simulink model "Guardian_Battery"  (R2025b)
settings: Solver=FixedStepDiscrete  StartTime=0.0  StopTime=T_end_s  FixedStep=Ts  RelTol=1e-3
model workspace (MAT data in the model file):
  TLS_impl_select = 2
values from neighbouring files (symbols this model uses):
  a1_coef = exp(-Ts/(tau1_s))    [Guardian_Battery_script.m]
  a2_coef = exp(-Ts/(tau2_s))    [Guardian_Battery_script.m]
  hyst_filt_den = [1, -a_hyst_coef]    [Guardian_Battery_script.m]
  hyst_filt_num = 1 - a_hyst_coef    (= 0.00201823135843)    [Guardian_Battery_script.m]
  OCV_data = ocvLookupTbl.OCV_V    [Guardian_Battery_script.m]
  Q_nominal = 50    [Guardian_Battery_script.m]
  R0_ref = 0.0007    [Guardian_Battery_script.m]
  R1_ref = 0.0016    [Guardian_Battery_script.m]
  R2_ref = 0.00035    [Guardian_Battery_script.m]
  SOC_breakpoints = ocvLookupTbl.SOC_pct    [Guardian_Battery_script.m]
  SOC_init_pct = 80    [Guardian_Battery_script.m]
  Ts = 0.1    [Guardian_Battery_script.m]
undefined symbols (not defined in the file or in its folder): DiscIntNeverNeededParam, dspblkCoreblockFVToolHelper, gcbh
libraries: simulink x2
settings Model: Creator=LENOVO  LastModifiedBy=Ahmed

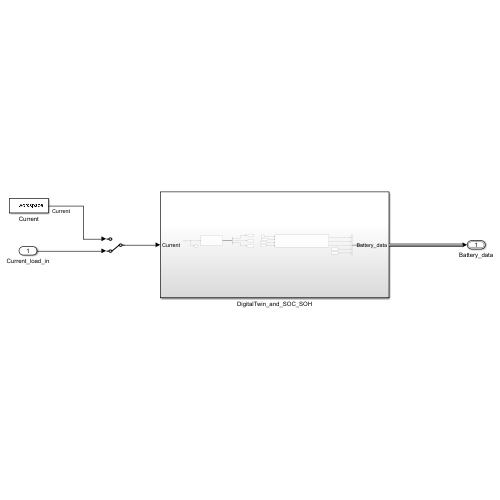
[thumbnail: Simulink's stored preview of the top-level diagram]
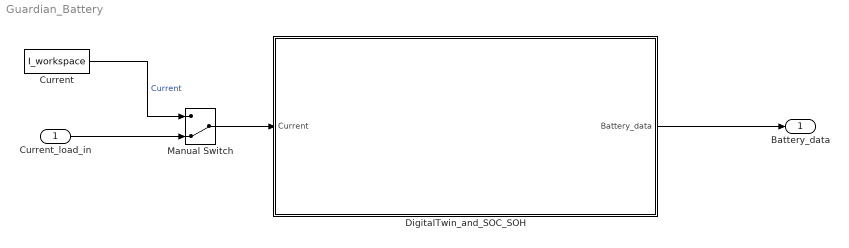
== system Guardian_Battery ==
  Current_load_in : Inport
  Current : FromWorkspace  VariableName=I_workspace
  DigitalTwin_and_SOC_SOH : Subsystem
  Manual Switch : ManualSwitch  CurrentSetting=0
  Battery_data : Outport  OutDataTypeStr=Bus: BatteryDataBus
  wires:
  DigitalTwin_and_SOC_SOH/1(Battery_data) -> Battery_data/1
  Current/1 -> Manual Switch/1  "Current"
  Manual Switch/1 -> DigitalTwin_and_SOC_SOH/1(Current)
  Current_load_in/1 -> Manual Switch/2

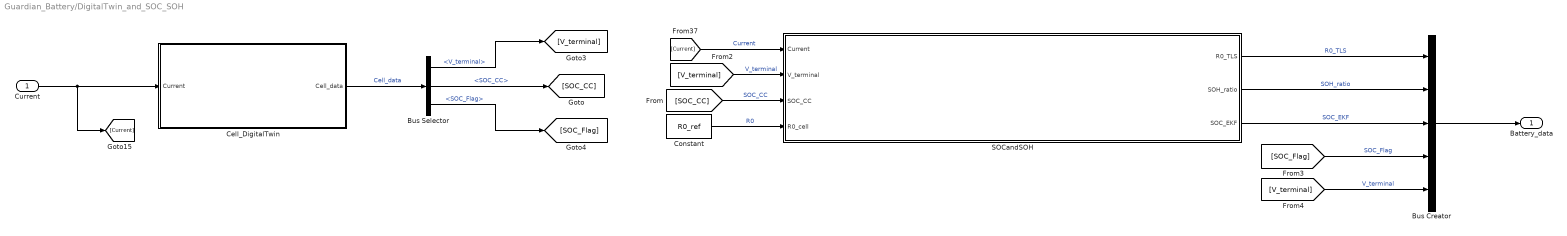
== system Guardian_Battery/DigitalTwin_and_SOC_SOH ==
  Current : Inport
  Bus Creator : BusCreator  Inputs=5  OutDataTypeStr=Bus: BatteryDataBus
  Bus Selector : BusSelector  OutputSignals=V_terminal,SOC_CC,SOC_Flag
  Cell_DigitalTwin : Subsystem
  Constant : Constant  Value=R0_ref
  SOCandSOH : Subsystem
  Battery_data : Outport  OutDataTypeStr=Bus: BatteryDataBus
  wires:
  Bus Selector/1 -> [V_terminal]  "<V_terminal>"
  Bus Selector/2 -> [SOC_CC]  "<SOC_CC>"
  Bus Selector/3 -> [SOC_Flag]  "<SOC_Flag>"
  Cell_DigitalTwin/1(Cell_data) -> Bus Selector/1  "Cell_data"
  Current/1 -> [Current], Cell_DigitalTwin/1(Current)
  [Current] -> SOCandSOH/1(Current)  "Current"
  [V_terminal] -> SOCandSOH/2(V_terminal)  "V_terminal"
  [SOC_CC] -> SOCandSOH/3(SOC_CC)  "SOC_CC"
  Constant/1 -> SOCandSOH/4(R0_cell)  "R0"
  SOCandSOH/1(R0_TLS) -> Bus Creator/1  "R0_TLS"
  SOCandSOH/2(SOH_ratio) -> Bus Creator/2  "SOH_ratio"
  SOCandSOH/3(SOC_EKF) -> Bus Creator/3  "SOC_EKF"
  [SOC_Flag] -> Bus Creator/4  "SOC_Flag"
  [V_terminal] -> Bus Creator/5  "V_terminal"
  Bus Creator/1 -> Battery_data/1

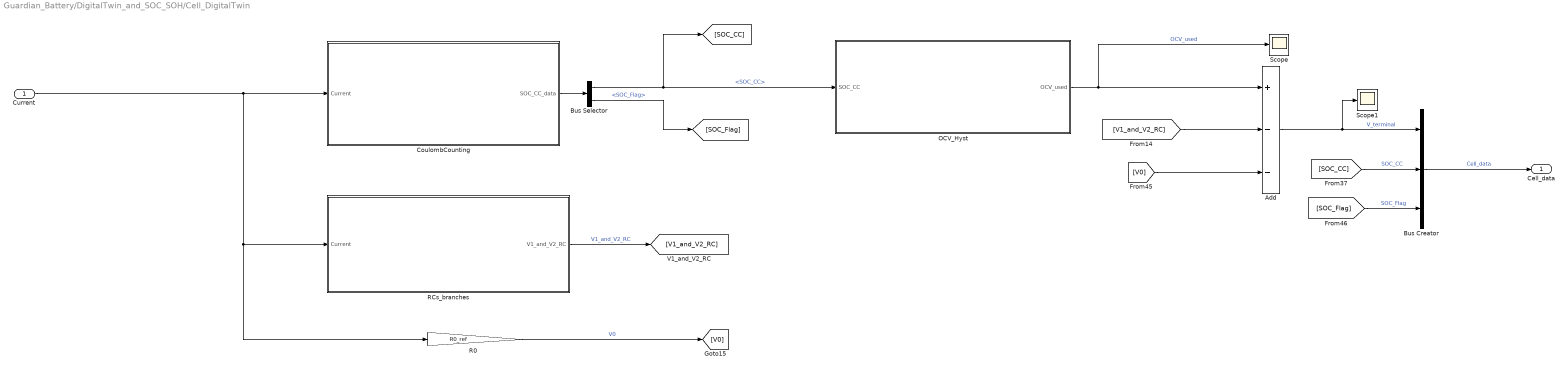
== system Guardian_Battery/DigitalTwin_and_SOC_SOH/Cell_DigitalTwin ==
  Current : Inport
  Add : Sum  Inputs=+--
  Bus Creator : BusCreator  Inputs=3
  Bus Selector : BusSelector  OutputSignals=SOC_CC,SOC_Flag
  CoulombCounting : Subsystem
  OCV_Hyst : Subsystem
  R0 : Gain  Gain=R0_ref
  RCs_branches : Subsystem
  Scope : Scope
  Scope1 : Scope
      settings: ActiveDisplayYMinimum=2.2986571776432272  ActiveDisplayYMaximum=4.2986571776432267  DataLoggingVariableName=ScopeData5
  Cell_data : Outport
  wires:
  Current/1 -> R0/1, RCs_branches/1(Current), CoulombCounting/1(Current)
  [V1_and_V2_RC] -> Add/2
  Bus Selector/2 -> [SOC_Flag]  "<SOC_Flag>"
  R0/1 -> [V0]  "V0"
  Bus Selector/1 -> [SOC_CC], OCV_Hyst/1(SOC_CC)  "<SOC_CC>"
  RCs_branches/1(V1_and_V2_RC) -> [V1_and_V2_RC]  "V1_and_V2_RC"
  OCV_Hyst/1(OCV_used) -> Scope/1, Add/1  "OCV_used"
  CoulombCounting/1(SOC_CC_data) -> Bus Selector/1
  [V0] -> Add/3
  Bus Creator/1 -> Cell_data/1  "Cell_data"
  [SOC_Flag] -> Bus Creator/3  "SOC_Flag"
  Add/1 -> Bus Creator/1, Scope1/1  "V_terminal"
  [SOC_CC] -> Bus Creator/2  "SOC_CC"

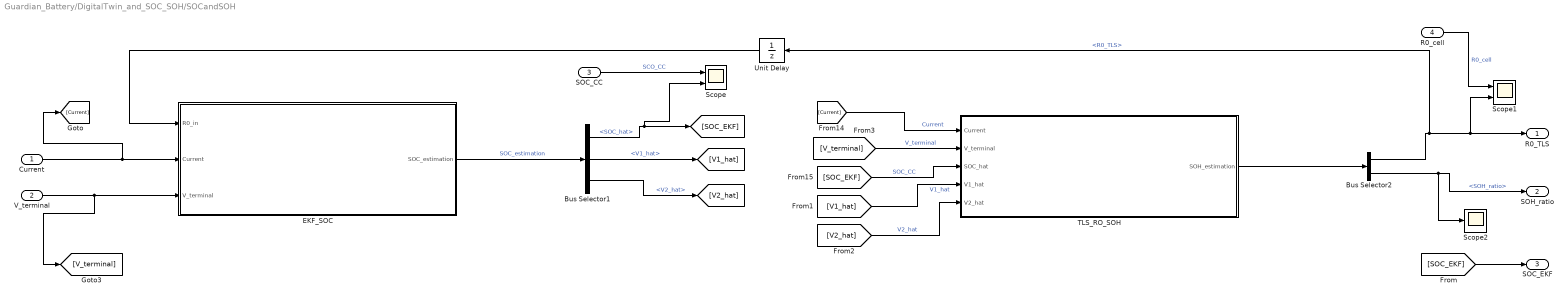
== system Guardian_Battery/DigitalTwin_and_SOC_SOH/SOCandSOH ==
  Current : Inport
  V_terminal : Inport  Port=2
  SOC_CC : Inport  Port=3
  R0_cell : Inport  Port=4
  Bus Selector1 : BusSelector  OutputSignals=SOC_hat,V1_hat,V2_hat
  Bus Selector2 : BusSelector  OutputSignals=R0_TLS,SOH_ratio
  EKF_SOC : Subsystem
  Scope : Scope  NumInputPorts=2
      settings: ActiveDisplayYMinimum=79.999123875594847  ActiveDisplayYMaximum=80.000097347156128  DataLoggingVariableName=ScopeData2
  Scope1 : Scope  NumInputPorts=2
      settings: ActiveDisplayYMinimum=0.00062720912057608426  ActiveDisplayYMaximum=0.000747148906633901  DataLoggingVariableName=ScopeData3
  Scope2 : Scope
      settings: ActiveDisplayYMinimum=93.43135778003041  ActiveDisplayYMaximum=111.29802568328962  DataLoggingVariableName=ScopeData4
  TLS_RO_SOH : Subsystem
  Unit Delay : UnitDelay  SampleTime=-1  HasFrameUpgradeWarning=on
  R0_TLS : Outport
  SOH_ratio : Outport  Port=2
  SOC_EKF : Outport  Port=3
  wires:
  [V_terminal] -> TLS_RO_SOH/2(V_terminal)  "V_terminal"
  TLS_RO_SOH/1(SOH_estimation) -> Bus Selector2/1
  [SOC_EKF] -> TLS_RO_SOH/3(SOC_hat)  "SOC_CC"
  Bus Selector1/2 -> [V1_hat]  "<V1_hat>"
  Bus Selector2/2 -> Scope2/1, SOH_ratio/1  "<SOH_ratio>"
  Bus Selector2/1 -> Scope1/2, R0_TLS/1, Unit Delay/1  "<R0_TLS>"
  Bus Selector1/1 -> Scope/2, [SOC_EKF]  "<SOC_hat>"
  EKF_SOC/1(SOC_estimation) -> Bus Selector1/1  "SOC_estimation"
  [Current] -> TLS_RO_SOH/1(Current)  "Current"
  V_terminal/1 -> [V_terminal], EKF_SOC/3(V_terminal)
  Current/1 -> [Current], EKF_SOC/2(Current)
  Bus Selector1/3 -> [V2_hat]  "<V2_hat>"
  [V1_hat] -> TLS_RO_SOH/4(V1_hat)  "V1_hat"
  [V2_hat] -> TLS_RO_SOH/5(V2_hat)  "V2_hat"
  Unit Delay/1 -> EKF_SOC/1(R0_in)
  SOC_CC/1 -> Scope/1  "SCO_CC"
  [SOC_EKF] -> SOC_EKF/1
  R0_cell/1 -> Scope1/1  "R0_cell"

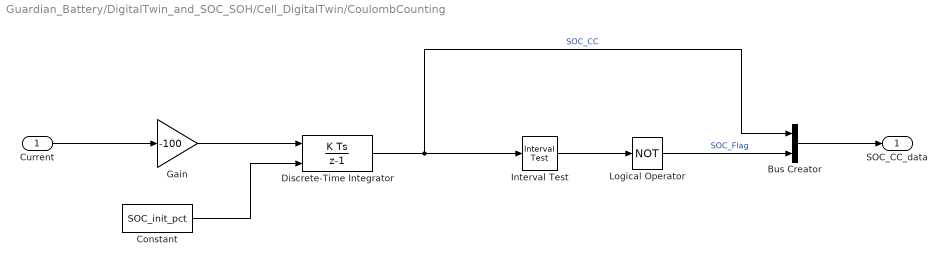
== system Guardian_Battery/DigitalTwin_and_SOC_SOH/Cell_DigitalTwin/CoulombCounting ==
  Current : Inport
  Bus Creator : BusCreator  Inputs=2
  Constant : Constant  Value=SOC_init_pct
  Discrete-Time Integrator : DiscreteIntegrator  gainval=1/(Q_nominal*3600)  InitialConditionSource=external  InitialCondition=80  SampleTime=Ts  LimitOutput=on  UpperSaturationLimit=90  LowerSaturationLimit=10  ICPrevOutput=DiscIntNeverNeededParam  ICPrevScaledInput=DiscIntNeverNeededParam
  Gain : Gain  Gain=-100
  Interval Test : simulink/Logic and Bit Operations/Interval Test  IntervalClosedRight=off  uplimit=90  IntervalClosedLeft=off  lowlimit=10  OutDataTypeStr=boolean
  Logical Operator : Logic  Operator=NOT  AllPortsSameDT=off  OutDataTypeStr=boolean
  SOC_CC_data : Outport
  wires:
  Current/1 -> Gain/1
  Gain/1 -> Discrete-Time Integrator/1
  Discrete-Time Integrator/1 -> Interval Test/1, Bus Creator/1  "SOC_CC"
  Logical Operator/1 -> Bus Creator/2  "SOC_Flag"
  Bus Creator/1 -> SOC_CC_data/1
  Constant/1 -> Discrete-Time Integrator/2
  Interval Test/1 -> Logical Operator/1

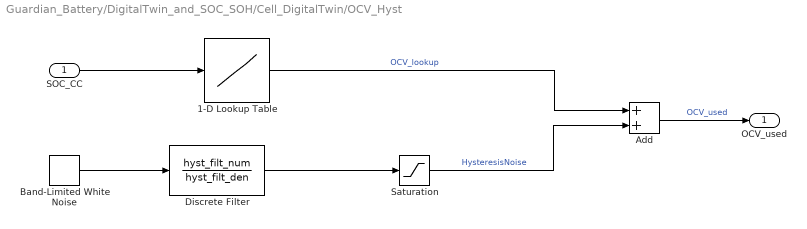
== system Guardian_Battery/DigitalTwin_and_SOC_SOH/Cell_DigitalTwin/OCV_Hyst ==
  SOC_CC : Inport
  1-D Lookup Table : Lookup_n-D  NumberOfTableDimensions=1  BreakpointsForDimension1=SOC_breakpoints  Table=OCV_data  ExtrapMethod=Clip  InternalRulePriority=Speed  RndMeth=Simplest
  Add : Sum
  Band-Limited White Noise : simulink/Sources/Band-Limited White Noise  Cov=[1e-4]  Ts=Ts  seed=[23341]
  Discrete Filter : DiscreteFilter  LoadFcn=dspblkCoreblockFVToolHelper(gcbh,'load');  Numerator=hyst_filt_num  Denominator=hyst_filt_den
      settings: CopyFcn=dspblkCoreblockFVToolHelper(gcbh,'copy');  DeleteFcn=dspblkCoreblockFVToolHelper(gcbh,'close');  ModelCloseFcn=dspblkCoreblockFVToolHelper(gcbh,'close');  PreSaveFcn=dspblkCoreblockFVToolHelper(gcbh,'presave');  PostSaveFcn=dspblkCoreblockFVToolHelper(gcbh,'postsave');  CloseFcn=dspblkCoreblockFVToolHelper(gcbh,'close');
  Saturation : Saturate  UpperLimit=0.005  LowerLimit=-0.005
  OCV_used : Outport
  wires:
  SOC_CC/1 -> 1-D Lookup Table/1
  1-D Lookup Table/1 -> Add/1  "OCV_lookup"
  Band-Limited White Noise/1 -> Discrete Filter/1
  Discrete Filter/1 -> Saturation/1
  Saturation/1 -> Add/2  "HysteresisNoise"
  Add/1 -> OCV_used/1  "OCV_used"

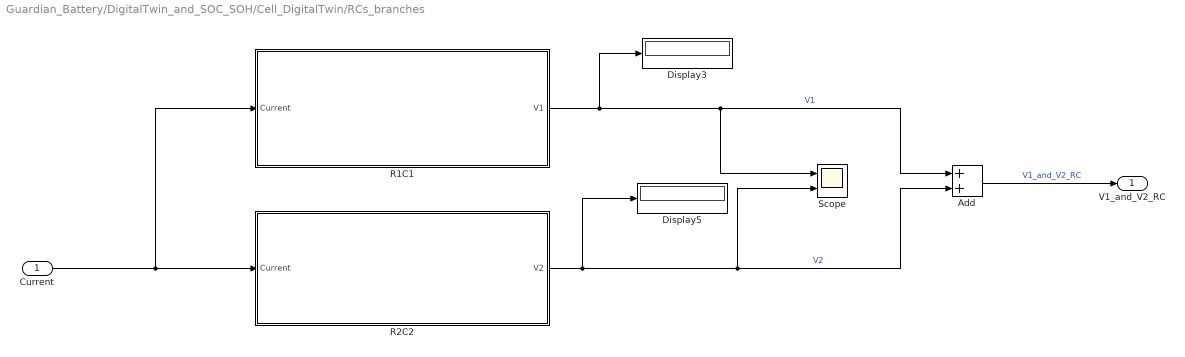
== system Guardian_Battery/DigitalTwin_and_SOC_SOH/Cell_DigitalTwin/RCs_branches ==
  Current : Inport
  Add : Sum
  Display3 : Display
  Display5 : Display
  R1C1 : Subsystem
  R2C2 : Subsystem
  Scope : Scope  NumInputPorts=2
  V1_and_V2_RC : Outport
  wires:
  Current/1 -> R2C2/1(Current), R1C1/1(Current)
  R1C1/1(V1) -> Add/1, Scope/1, Display3/1  "V1"
  R2C2/1(V2) -> Add/2, Scope/2, Display5/1  "V2"
  Add/1 -> V1_and_V2_RC/1  "V1_and_V2_RC"

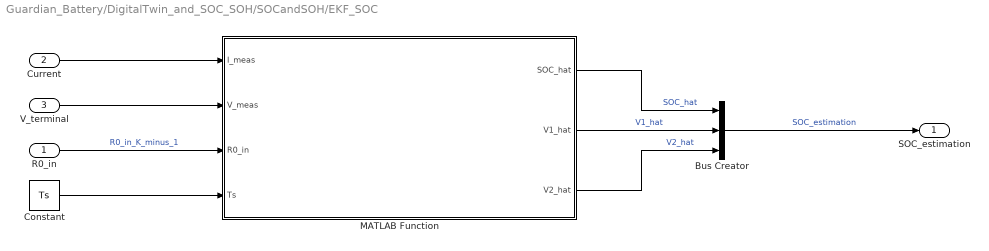
== system Guardian_Battery/DigitalTwin_and_SOC_SOH/SOCandSOH/EKF_SOC ==
  R0_in : Inport
  Current : Inport  Port=2
  V_terminal : Inport  Port=3
  Bus Creator : BusCreator  Inputs=3
  Constant : Constant  Value=Ts
  MATLAB Function : MATLAB Function  TreatAsAtomicUnit=on
  SOC_estimation : Outport
  wires:
  Current/1 -> MATLAB Function/1(I_meas)
  V_terminal/1 -> MATLAB Function/2(V_meas)
  Constant/1 -> MATLAB Function/4(Ts)
  MATLAB Function/1(SOC_hat) -> Bus Creator/1  "SOC_hat"
  MATLAB Function/2(V1_hat) -> Bus Creator/2  "V1_hat"
  Bus Creator/1 -> SOC_estimation/1  "SOC_estimation"
  MATLAB Function/3(V2_hat) -> Bus Creator/3  "V2_hat"
  R0_in/1 -> MATLAB Function/3(R0_in)  "R0_in_K_minus_1"

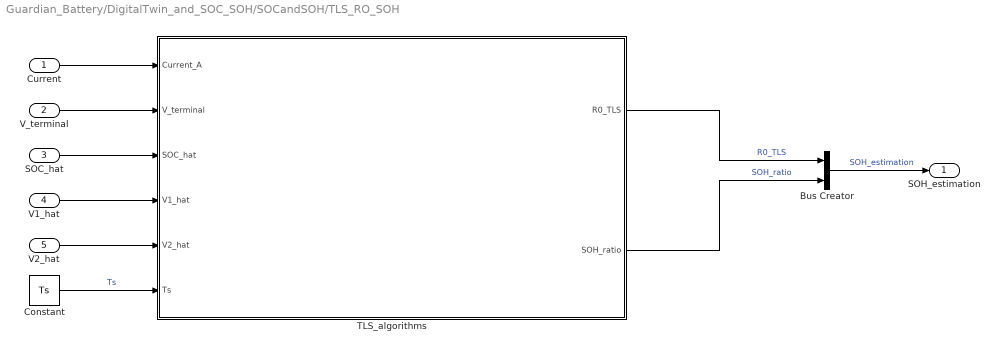
== system Guardian_Battery/DigitalTwin_and_SOC_SOH/SOCandSOH/TLS_RO_SOH ==
  Current : Inport
  V_terminal : Inport  Port=2
  SOC_hat : Inport  Port=3
  V1_hat : Inport  Port=4
  V2_hat : Inport  Port=5
  Bus Creator : BusCreator  Inputs=2
  Constant : Constant  Value=Ts
  TLS_algorithms : Subsystem  Variant=on  EmptyChoice=on
  SOH_estimation : Outport
  wires:
  Bus Creator/1 -> SOH_estimation/1  "SOH_estimation"
  Current/1 -> TLS_algorithms/1(Current_A)
  V_terminal/1 -> TLS_algorithms/2(V_terminal)
  SOC_hat/1 -> TLS_algorithms/3(SOC_hat)
  V1_hat/1 -> TLS_algorithms/4(V1_hat)
  V2_hat/1 -> TLS_algorithms/5(V2_hat)
  Constant/1 -> TLS_algorithms/6(Ts)  "Ts"
  TLS_algorithms/1(R0_TLS) -> Bus Creator/1  "R0_TLS"
  TLS_algorithms/2(SOH_ratio) -> Bus Creator/2  "SOH_ratio"

== system Guardian_Battery/DigitalTwin_and_SOC_SOH/Cell_DigitalTwin/RCs_branches/R1C1 ==
  Current : Inport
  Add : Sum
  Gain : Gain  Gain=R1_ref * (1-a1_coef)
  Gain1 : Gain  Gain=a1_coef
  Unit Delay : UnitDelay  SampleTime=-1  HasFrameUpgradeWarning=on
  V1 : Outport
  wires:
  Current/1 -> Gain/1
  Gain/1 -> Add/1
  Add/1 -> Unit Delay/1
  Unit Delay/1 -> Gain1/1, V1/1  "V1"
  Gain1/1 -> Add/2

== system Guardian_Battery/DigitalTwin_and_SOC_SOH/Cell_DigitalTwin/RCs_branches/R2C2 ==
  Current : Inport
  Add : Sum
  Gain : Gain  Gain=R2_ref * (1 - a2_coef)
  Gain1 : Gain  Gain=a2_coef
  Unit Delay : UnitDelay  SampleTime=-1  HasFrameUpgradeWarning=on
  V2 : Outport
  wires:
  Current/1 -> Gain/1
  Gain/1 -> Add/1
  Add/1 -> Unit Delay/1
  Unit Delay/1 -> Gain1/1, V2/1  "V2"
  Gain1/1 -> Add/2

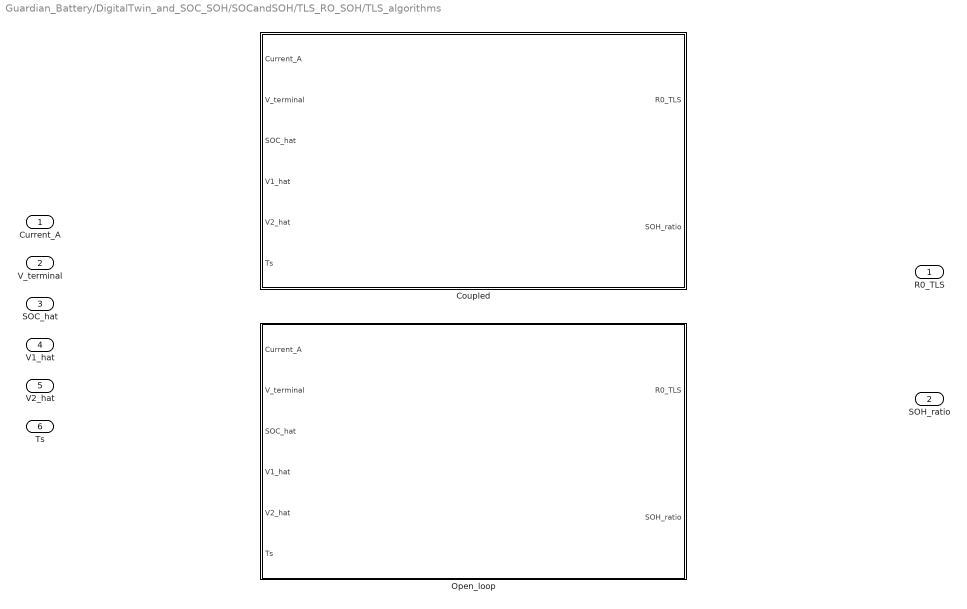
== system Guardian_Battery/DigitalTwin_and_SOC_SOH/SOCandSOH/TLS_RO_SOH/TLS_algorithms ==
  Current_A : Inport
  V_terminal : Inport  Port=2
  SOC_hat : Inport  Port=3
  V1_hat : Inport  Port=4
  V2_hat : Inport  Port=5
  Ts : Inport  Port=6
  Coupled : Subsystem  VariantControl=TLS_impl_select == 1
  Open_loop : Subsystem  VariantControl=TLS_impl_select == 2
  R0_TLS : Outport
  SOH_ratio : Outport  Port=2

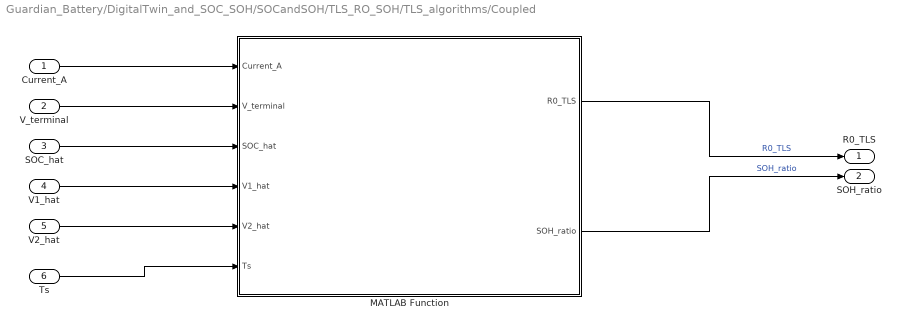
== system Guardian_Battery/DigitalTwin_and_SOC_SOH/SOCandSOH/TLS_RO_SOH/TLS_algorithms/Coupled ==
  Current_A : Inport
  V_terminal : Inport  Port=2
  SOC_hat : Inport  Port=3
  V1_hat : Inport  Port=4
  V2_hat : Inport  Port=5
  Ts : Inport  Port=6
  MATLAB Function : MATLAB Function  TreatAsAtomicUnit=on
  R0_TLS : Outport
  SOH_ratio : Outport  Port=2
  wires:
  SOC_hat/1 -> MATLAB Function/3(SOC_hat)
  MATLAB Function/2(SOH_ratio) -> SOH_ratio/1  "SOH_ratio"
  MATLAB Function/1(R0_TLS) -> R0_TLS/1  "R0_TLS"
  Current_A/1 -> MATLAB Function/1(Current_A)
  Ts/1 -> MATLAB Function/6(Ts)
  V2_hat/1 -> MATLAB Function/5(V2_hat)
  V_terminal/1 -> MATLAB Function/2(V_terminal)
  V1_hat/1 -> MATLAB Function/4(V1_hat)

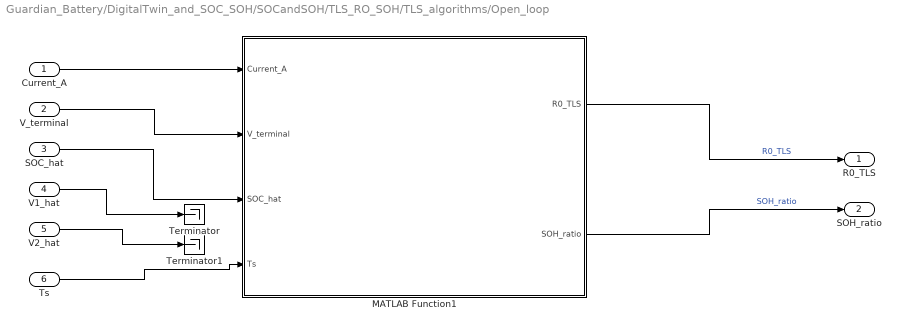
== system Guardian_Battery/DigitalTwin_and_SOC_SOH/SOCandSOH/TLS_RO_SOH/TLS_algorithms/Open_loop ==
  Current_A : Inport
  V_terminal : Inport  Port=2
  SOC_hat : Inport  Port=3
  V1_hat : Inport  Port=4
  V2_hat : Inport  Port=5
  Ts : Inport  Port=6
  MATLAB Function1 : MATLAB Function  TreatAsAtomicUnit=on
  Terminator : Terminator
  Terminator1 : Terminator
  R0_TLS : Outport
  SOH_ratio : Outport  Port=2
  wires:
  V1_hat/1 -> Terminator/1
  V_terminal/1 -> MATLAB Function1/2(V_terminal)
  V2_hat/1 -> Terminator1/1
  Ts/1 -> MATLAB Function1/4(Ts)
  Current_A/1 -> MATLAB Function1/1(Current_A)
  MATLAB Function1/1(R0_TLS) -> R0_TLS/1  "R0_TLS"
  MATLAB Function1/2(SOH_ratio) -> SOH_ratio/1  "SOH_ratio"
  SOC_hat/1 -> MATLAB Function1/3(SOC_hat)

== matlab function Guardian_Battery/DigitalTwin_and_SOC_SOH/SOCandSOH/TLS_RO_SOH/TLS_algorithms/Coupled/MATLAB Function ==
  data: Current_A input; R0_TLS output; V_terminal input; SOC_hat input; SOH_ratio output; V1_hat input; V2_hat input; Ts input
function [R0_TLS, SOH_ratio] = TLS_RO_SOH_block(Current_A, V_terminal, SOC_hat, V1_hat, V2_hat, Ts)
%TLS_RO_SOH_BLOCK  Recursive (online) TLS identification of R0, closing
%   the loop with the EKF -- Part 2 Addendum to Sec. 6.5 / Figure 4.
%
%   [R0_TLS, SOH_ratio] = TLS_RO_SOH_block(Current_A, V_terminal, ...
%                                            SOC_hat, V1_hat, V2_hat, Ts)
%
%   Inputs:
%     Current_A   - measured cell current (A), discharge = POSITIVE
%     V_terminal  - measured/simulated terminal voltage (V)
%     SOC_hat     - EKF's SOC estimate (%) -- replaces SOC_CC from the
%                   original spec so TLS regresses against the same
%                   state the EKF tracks, not the open-loop CC value
%     V1_hat      - EKF's R1C1 polarization estimate (V) -- replaces
%                   this block's own open-loop V1 computation
%     V2_hat      - EKF's R2C2 polarization estimate (V)
%     Ts          - sample time (s)
%
%   Outputs:
%     R0_TLS      - live R0 estimate (ohm), rate-limited (held) before
%                   being sent to the EKF -- see updateEvery below.
%                   Feed this into EKF_SOC_Estimator's R0_in through a
%                   Unit Delay/Memory block, not directly.
%     SOH_ratio   - R0_datasheet / R0_TLS * 100 (%)
%
%   COUPLING NOTE: because V1_hat/V2_hat now come from the same EKF that
%   R0_TLS feeds, an R0 error partially gets absorbed into the EKF's own
%   correction step rather than showing up cleanly as residual here.
%   updateEvery decouples the two update rates (recursive stats refresh
%   every sample; the value actually pushed to the EKF refreshes every
%   updateEvery samples) so the EKF has time to resettle between R0
%   pushes. Set updateEvery = 1 to disable this and go fully tight-
%   coupled if you'd rather observe that behavior directly.
%#codegen
persistent mx my Sxx Sxy Syy R0_running R0_held sampleCount initialized

R0_nominal = 0.00070;   % datasheet R0 (ohm) -- seed value + fallback

if isempty(initialized)
    mx = 0; my = 0; Sxx = 0; Sxy = 0; Syy = 0;
    R0_running  = R0_nominal;
    R0_held     = R0_nominal;
    sampleCount = 0;
    initialized = true;
end

soc_bp = [0 5 10 20 30 40 50 60 70 80 90 95 100];
ocv_bp = [2.50 2.95 3.05 3.15 3.20 3.22 3.24 3.26 3.28 3.30 3.33 3.45 3.65];

% lambda was originally tuned at Ts_ref=1 (tau ~= 333 s real-time memory).
% Rescaled here the same way as hyst_num/hyst_den in the main script --
% left unscaled, Ts=0.1 would silently shrink the memory window to ~33 s,
% making the estimator far more sensitive to short poorly-conditioned
% stretches of data (this was the cause of the R0_TLS transient spikes).
Ts_ref_lambda = 1;
lambda_ref    = 0.997;
lambda        = lambda_ref ^ (Ts / Ts_ref_lambda);
minSxx      = 1e-4;                % persistent-excitation guard
minSxyAbs   = 1e-8;
updateEvery = max(1, round(5/Ts)); % push a new R0 to the EKF ~every 5 s
R0_min      = 0.1 * R0_nominal;    % physical-plausibility guard --
R0_max      = 5   * R0_nominal;    % reject candidates outside a sane range

% ---- regression target/regressor, per Sec. 6.5, now sourced from the EKF ----
OCV_k = interp1(soc_bp, ocv_bp, SOC_hat, 'linear', 'extrap');
y_k = OCV_k - V1_hat - V2_hat - V_terminal;
x_k = Current_A;

% ---- recursive (exponentially-weighted) TLS update -----------------------
mx = lambda*mx + (1-lambda)*x_k;
my = lambda*my + (1-lambda)*y_k;
dx = x_k - mx;
dy = y_k - my;

Sxx = lambda*Sxx + (1-lambda)*dx^2;
Sxy = lambda*Sxy + (1-lambda)*dx*dy;
Syy = lambda*Syy + (1-lambda)*dy^2;

if Sxx > minSxx && abs(Sxy) > minSxyAbs
    D = (Sxx - Syy)^2 + 4*Sxy^2;
    R0_candidate = ((Syy - Sxx) + sqrt(D)) / (2*Sxy);  % == -V(1,2)/V(2,2) from the batch SVD form
    if R0_candidate > R0_min && R0_candidate < R0_max
        R0_running = R0_candidate;
    end
    % else: reject as physically implausible, keep the last good R0_running
end

% ---- rate-limit the value actually pushed to the EKF ---------------------
sampleCount = sampleCount + 1;
if sampleCount >= updateEvery
    R0_held = R0_running;
    sampleCount = 0;
end

R0_TLS    = R0_held;
SOH_ratio = (R0_nominal / R0_TLS) * 100;
end

== matlab function Guardian_Battery/DigitalTwin_and_SOC_SOH/SOCandSOH/EKF_SOC/MATLAB Function ==
  data: I_meas input; SOC_hat output; V_meas input; R0_in input; Ts input; V1_hat output; V2_hat output
function [SOC_hat, V1_hat, V2_hat] = EKF_SOC_Estimator(I_meas, V_meas, R0_in, Ts)
%EKF_SOC_ESTIMATOR  Extended Kalman Filter SOC estimator for the Guardian
%   Battery ECM Project (2RC Thevenin model, LF50K 3.2V/50Ah LFP cell).
%
%   [SOC_hat, V1_hat, V2_hat] = EKF_SOC_Estimator(I_meas, V_meas, R0_in, Ts)
%
%   Inputs:
%     I_meas  - measured cell current (A), discharge = POSITIVE
%     V_meas  - measured terminal voltage (V)
%     R0_in   - live R0 estimate (ohm), fed from TLS_RO_SOH_block, ONE
%               SAMPLE DELAYED (put a Unit Delay/Memory block on this
%               wire in Simulink) -- R0 is no longer a fixed constant
%     Ts      - sample time (s) -- must match the model's discrete step
%
%   Outputs:
%     SOC_hat - estimated state of charge (%)
%     V1_hat  - estimated R1C1-branch polarization voltage (V)
%     V2_hat  - estimated R2C2-branch polarization voltage (V)
%
%   Part 2 Addendum: extended from 1RC/2-state to 2RC/3-state, and R0
%   promoted from a fixed constant to a live input from the recursive
%   TLS identifier -- this closes the joint state/parameter estimation
%   loop with TLS_RO_SOH_block.m.
%#codegen
persistent x P initialized
if isempty(initialized)
    x = [80; 0; 0];               % [SOC(%); V1(V); V2(V)]
    P = diag([4, 0.01, 0.01]);    % initial covariance
    initialized = true;
end

% ---- Fixed cell/model parameters (from project datasheet, Appendix A) ----
Q_nominal_Ah = 50;
R1 = 0.00160;      % ohm
C1 = 17000;        % F
R2 = 0.00035;      % ohm
C2 = 5200;         % F
a1 = exp(-Ts / (R1*C1));
a2 = exp(-Ts / (R2*C2));

% ---- OCV-SOC breakpoints -- MUST match Guardian_Battery_OCV_SOC_Table.csv ----
soc_bp = [0 5 10 20 30 40 50 60 70 80 90 95 100];
ocv_bp = [2.50 2.95 3.05 3.15 3.20 3.22 3.24 3.26 3.28 3.30 3.33 3.45 3.65];

% ---- Process/measurement noise tuning ----
% Qcov was originally tuned at Ts_ref = 1 s. Discrete process noise
% accumulates roughly linearly with Ts (more, smaller steps per second
% should inject proportionally less noise per step to match the same
% real-time uncertainty growth) -- scaled here, but still a starting
% point to retune/justify like the original two entries were.
Ts_ref = 1;
Qcov = diag([1e-3, 1e-6, 1e-6]) * (Ts / Ts_ref);
Rcov = 4e-4;   % sensor noise -- not Ts-dependent, left as-is

% =====================================================================
% PREDICT
% =====================================================================
SOC_pred = x(1) - (Ts / (Q_nominal_Ah * 3600)) * I_meas * 100;
V1_pred  = a1 * x(2) + R1 * (1 - a1) * I_meas;
V2_pred  = a2 * x(3) + R2 * (1 - a2) * I_meas;
x_pred = [SOC_pred; V1_pred; V2_pred];

F = [1, 0,  0;
     0, a1, 0;
     0, 0,  a2];
P_pred = F * P * F' + Qcov;

% =====================================================================
% UPDATE
% =====================================================================
OCV_pred  = interp1(soc_bp, ocv_bp, x_pred(1), 'linear', 'extrap');
d = 0.5;
dOCV_dSOC = interp1(soc_bp, ocv_bp, x_pred(1) + d, 'linear', 'extrap') ...
          - interp1(soc_bp, ocv_bp, x_pred(1) - d, 'linear', 'extrap');
dOCV_dSOC = dOCV_dSOC / (2 * d);

H = [dOCV_dSOC, -1, -1];
V_pred = OCV_pred - I_meas * R0_in - x_pred(2) - x_pred(3);
y_resid = V_meas - V_pred;
S = H * P_pred * H' + Rcov;
K = P_pred * H' / S;
x = x_pred + K * y_resid;
P = (eye(3) - K * H) * P_pred;

% Physical bound -- SOC cannot leave [0, 100]%
x(1) = min(max(x(1), 0), 100);

SOC_hat = x(1);
V1_hat  = x(2);
V2_hat  = x(3);
end

== matlab function Guardian_Battery/DigitalTwin_and_SOC_SOH/SOCandSOH/TLS_RO_SOH/TLS_algorithms/Open_loop/MATLAB Function1 ==
  data: Current_A input; R0_TLS output; V_terminal input; SOC_hat input; SOH_ratio output; Ts input
function [R0_TLS, SOH_ratio] = TLS_RO_SOH_block_openloop(Current_A, V_terminal, SOC_hat, Ts)
%TLS_RO_SOH_BLOCK_OPENLOOP  Recursive (online) TLS identification of R0,
%   using OPEN-LOOP V1/V2 computed from the GIVEN R1,C1,R2,C2 -- per
%   spec Sec. 6.5's original design intent ("skipping this step biases
%   the R0 estimate significantly"), rather than the EKF's own V1_hat/
%   V2_hat. Only R0_TLS feeds back into the EKF (one-way coupling);
%   this block's own RC-branch replica is independent of the EKF's
%   real-time estimation error, so an EKF transient can't leak into
%   the R0 regression residual.
%
%   [R0_TLS, SOH_ratio] = TLS_RO_SOH_block_openloop(Current_A, ...
%                                            V_terminal, SOC_hat, Ts)
%
%   Inputs:
%     Current_A   - measured cell current (A), discharge = POSITIVE
%     V_terminal  - measured/simulated terminal voltage (V)
%     SOC_hat     - EKF's SOC estimate (%)
%     Ts          - sample time (s)
%
%   Outputs:
%     R0_TLS      - live R0 estimate (ohm), rate-limited (held) before
%                   being sent to the EKF -- see updateEvery below.
%                   Feed into EKF_SOC_Estimator's R0_in through a Unit
%                   Delay/Memory block, same wiring as the coupled
%                   version. Note this block no longer takes V1_hat/
%                   V2_hat as inputs -- two fewer ports than before.
%     SOH_ratio   - R0_datasheet / R0_TLS * 100 (%)
%#codegen
persistent mx my Sxx Sxy Syy R0_running R0_held sampleCount V1_ol V2_ol initialized

R0_nominal = 0.00070;   % datasheet R0 (ohm) -- seed value + fallback
R1 = 0.00160;      % ohm -- GIVEN, known (not estimated here)
C1 = 17000;        % F
R2 = 0.00035;      % ohm
C2 = 5200;         % F

if isempty(initialized)
    mx = 0; my = 0; Sxx = 0; Sxy = 0; Syy = 0;
    R0_running  = R0_nominal;
    R0_held     = R0_nominal;
    sampleCount = 0;
    V1_ol = 0;   % battery assumed at rest, no polarization, at t=0
    V2_ol = 0;
    initialized = true;
end

soc_bp = [0 5 10 20 30 40 50 60 70 80 90 95 100];
ocv_bp = [2.50 2.95 3.05 3.15 3.20 3.22 3.24 3.26 3.28 3.30 3.33 3.45 3.65];

a1 = exp(-Ts/(R1*C1));
a2 = exp(-Ts/(R2*C2));

% lambda scaled the same way as the coupled version -- see that file's
% comment for why this matters at Ts != 1.
Ts_ref_lambda = 1;
lambda_ref    = 0.997;
lambda        = lambda_ref ^ (Ts / Ts_ref_lambda);
minSxx      = 1e-4;                % persistent-excitation guard
minSxyAbs   = 1e-8;
updateEvery = max(1, round(5/Ts)); % push a new R0 to the EKF ~every 5 s
R0_min      = 0.1 * R0_nominal;    % physical-plausibility guard
R0_max      = 5   * R0_nominal;

% ---- regression target/regressor, per Sec. 6.5, OPEN-LOOP V1/V2 ---------
% NOTE: uses V1_ol(k)/V2_ol(k), i.e. the values BEFORE this step's
% advance, matching the index convention in Sec. 6.5.
OCV_k = interp1(soc_bp, ocv_bp, SOC_hat, 'linear', 'extrap');
y_k = OCV_k - V1_ol - V2_ol - V_terminal;
x_k = Current_A;

% ---- THEN advance the open-loop RC replica, given R1,C1,R2,C2 ----------
V1_ol = a1*V1_ol + R1*(1-a1)*Current_A;
V2_ol = a2*V2_ol + R2*(1-a2)*Current_A;

% ---- recursive (exponentially-weighted) TLS update -----------------------
mx = lambda*mx + (1-lambda)*x_k;
my = lambda*my + (1-lambda)*y_k;
dx = x_k - mx;
dy = y_k - my;

Sxx = lambda*Sxx + (1-lambda)*dx^2;
Sxy = lambda*Sxy + (1-lambda)*dx*dy;
Syy = lambda*Syy + (1-lambda)*dy^2;

if Sxx > minSxx && abs(Sxy) > minSxyAbs
    D = (Sxx - Syy)^2 + 4*Sxy^2;
    R0_candidate = ((Syy - Sxx) + sqrt(D)) / (2*Sxy);  % == -V(1,2)/V(2,2) from the batch SVD form
    if R0_candidate > R0_min && R0_candidate < R0_max
        R0_running = R0_candidate;
    end
    % else: reject as physically implausible, keep the last good R0_running
end

% ---- rate-limit the value actually pushed to the EKF ---------------------
sampleCount = sampleCount + 1;
if sampleCount >= updateEvery
    R0_held = R0_running;
    sampleCount = 0;
end

R0_TLS    = R0_held;
SOH_ratio = (R0_nominal / R0_TLS) * 100;
end
